simulink model "MyRhoVar"  (Simulink 7.9)
settings: Solver=FixedStepDiscrete  StartTime=0.0  StopTime=1e8  FixedStep=1  RelTol=1e-3
(part 1 of 3)
settings Model: Creator=awohlfei  LastModifiedBy=awohlfei
settings DataIOCC: SaveTime=off
settings SFSimCC: SimUserSources=carlib.c

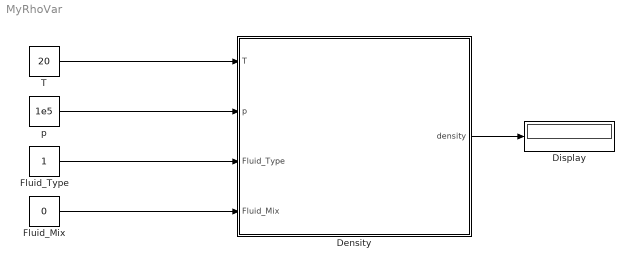
== system MyRhoVar ==
  Density : Subsystem  Variant=on  OverrideUsingVariant=CarlibWithErrorManagement1  mask{CALCMETHOD=CarlibWithErrorManagement1, INPUTARGUMENTS=state variables (classic), DEBUGLEVEL=ERROR, MAXTOTALWARNINGS=inf, MAXCONSECUTIVEWARNINGS=inf, WRITETOFILE=0, FILENAME='m.txt', TLOOKUP=[0 100], PLOOKUP=[0.5 5]*1e5, MIXLOOKUP=[0 1], DENSITYLOOKUP=ones(2,2,2)*1000, POLYNOMIALCOEFFICIENTS=[-0.003564 -0.07696 1001.0], CONSTANTVALUE=1000.0}
      mask prompts: CALCMETHOD "Calculation method"; INPUTARGUMENTS "Input arguments"
      mask init:
      | CalcmethodString=get_param(gcb,'CALCMETHOD');
      | 
      | UNUSEDINPORTS={}; %initialisation necessary, otherwise the active variant does not have this parameter in the next step (this is important for running the model)
      | 
      | %set choosen variant active
      | set_param([gcb,'/',CalcmethodString],'ACTIVE','1');
      | if str2num(get_param([gcb,'/',CalcmethodString],'DUMMY'))==0 %change in the flag ensures execution of the initialisation commands
      |     set_param([gcb,'/',CalcmethodString],'DUMMY','1');
      | else
      |     set_param([gcb,'/',CalcmethodString],'DUMMY','0');
      | end
      | 
      | %read inports from the active variant
      | InportsActiveVariant=find_system([gcb,'/',CalcmethodString],'LookUnderMasks','all','FollowLinks','on','SearchDepth',1,'BlockType','Inport');
      | %read inports of teh variant subsystem
      | InportsParent=find_system(gcb,'LookUnderMasks','all','FollowLinks','on','SearchDepth',1,'BlockType','Inport');
      | %read all subsystems
      | SystemsPartent=find_system(gcb,'LookUnderMasks','all','FollowLinks','on','SearchDepth',1,'Variants','AllVariants','Blocktype','SubSystem');
      | 
      | 
      | %delete all unused ports
      | for CountParent=numel(InportsActiveVariant)+1:numel(InportsParent)
      |     delete_block(InportsParent{CountParent});
      | end
      | 
      | %rename / add inports
      | UNUSEDINPORTS=cell(numel(InportsActiveVariant),1);
      | for CountParent=1:numel(InportsActiveVariant)
      |     InportName=InportsActiveVariant{CountParent};
      |     SlashPos=strfind(InportName,'/');
      |     InportName=InportName(SlashPos(end)+1:end);
      |     UNUSEDINPORTS{CountParent}=InportName;
      |     if CountParent<=numel(InportsParent)
      |         set_param(InportsParent{CountParent},'Name',InportName);
      |     else
      |         add_block('built-in/Inport',[gcb,'/',InportName]);
      |     end
      |     set_param([gcb,'/',InportName],'Position',[55 100+50*CountParent 85 100+50*CountParent+14]);
      | end
      | 
      | %set all variants passive except the choosen one
      | for CountParent=2:numel(SystemsPartent) %element 1 is the name of the variant subsystem
      |     SysName=SystemsPartent{CountParent};
      |     SlashPos=strfind(SysName,'/');
      |     SysName=SysName(SlashPos(end)+1:end);
      |     if ~strcmp(SysName,CalcmethodString); %not the active one
      |         set_param(SystemsPartent{CountParent},'ACTIVE','0');
      |         if str2num(get_param(SystemsPartent{CountParent},'DUMMY'))==0 %change in the flag ensures execution of the initialisation commands
      |             set_param(SystemsPartent{CountParent},'DUMMY','1');
      |         else
      |             set_param(SystemsPartent{CountParent},'DUMMY','0');
      |         end
      |     end
      | end
      mask StyleString: popup(CarlibClassic|CarlibWithErrorManagement|CarlibWithErrorManagement1|Lookup|Polynomial|ConstantValue),popup(state variables (classic)|state variables (reduced)|THV|THB),popup(DEBUG|INFO|WARNING|ERROR|FATAL),edit,edit,edit,edit,edit,edit,edit,edit,edit,edit
      mask CallbackString:
      | set_param(gcb,'OverrideUsingVariant',get_param(gcb,'CALCMETHOD'));
      | switch get_param(gcb,'CALCMETHOD')
      |     case 'CarlibClassic'
      |         set_param(gcb,'MaskVisibilities',{'on','on','off','off','off','off','off','off','off','off','off','off','off'});
      |     case 'CarlibWithErrorManagement'
      |         set_param(gcb,'MaskVisibilities',{'on','on','on','on','on','on','on','off','off','off','off','off','off'});
      |     case 'CarlibWithErrorManagement1'
      |         set_param(gcb,'MaskVisibilities',{'on','on','on','on','on','on','on','off','off','off','off','off','off'});
      |     case 'Lookup'
      |         set_param(gcb,'MaskVisibilities',{'on','on','off','off','off','off','off','on','on','on','on','off','off'});
      |     case 'Polynomial'
      |         set_param(gcb,'MaskVisibilities',{'on','on','off','off','off','off','off','off','off','off','off','on','off'});
      |     case 'ConstantValue'
      |         set_param(gcb,'MaskVisibilities',{'on','on','off','off','off','off','off','off','off','off','off','off','on'});
      | end
      | ||||||||||||
  Display : Display
  Fluid_Mix : Constant  Value=0
  Fluid_Type : Constant
  T : Constant  Value=20
  p : Constant  Value=1e5
  wires:
  Density/1(density) -> Display/1
  p/1 -> Density/2(p)
  Fluid_Type/1 -> Density/3(Fluid_Type)
  Fluid_Mix/1 -> Density/4(Fluid_Mix)
  T/1 -> Density/1(T)
